simulink model "couplage_simulation"  (R2020a)
settings: Solver=VariableStepAuto  StartTime=0.0  StopTime=7  RelTol=1e-3
values from neighbouring files (symbols this model uses):
  cond_ini = [10; 10; 10; 0]    [bras.m]    (also in bras_espace.m = [10; 10; 10; 30]; bras_init.m = [10; 10; 10; 30]; init_simulation_couplage.m = [-pi/4; pi/4; -pi/4; 0])
  couples = [0; 0; 0; 0]    [init_simulation_couplage.m]
  inertie = [10; 10; 10]    [init_simulation_couplage.m]
  inertie_a = [0 0 0 0; 0 0 0 0; 0 0 0 0; 0 0 0 0]    [init_simulation_couplage.m]
  parametres = [m1; m2; m3; L1; L2; L3; l1; l2; l3; L0]    [init_simulation_couplage.m]
settings Model: Creator=loloche  LastModifiedBy=loloche

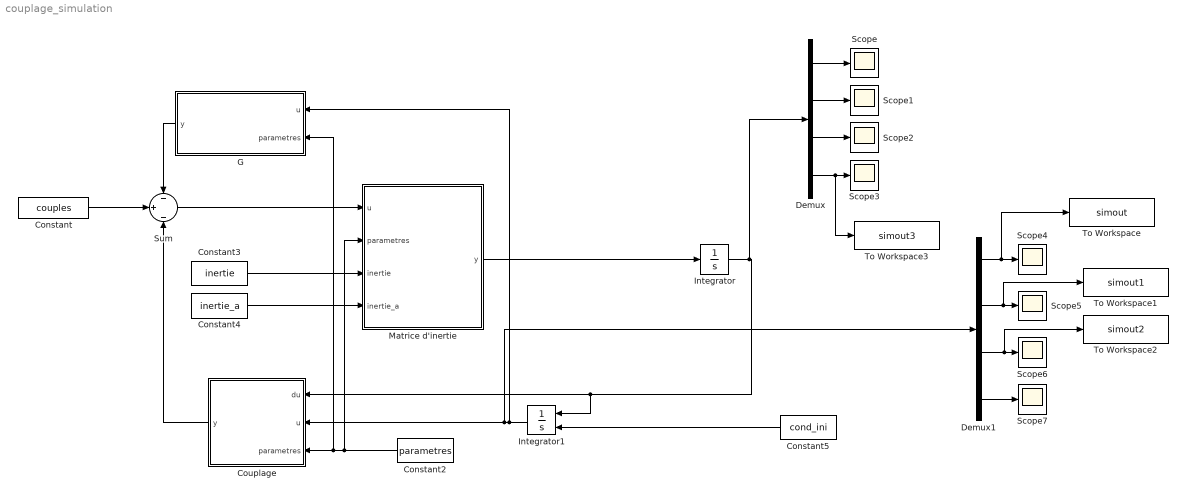
== system couplage_simulation ==
  Constant : Constant  Value=couples
  Constant2 : Constant  Value=parametres
  Constant3 : Constant  Value=inertie
  Constant4 : Constant  Value=inertie_a
  Constant5 : Constant  Value=cond_ini
  Couplage : MATLAB Function  TreatAsAtomicUnit=on
  Demux : Demux
  Demux1 : Demux
  G : MATLAB Function  TreatAsAtomicUnit=on
  Integrator : Integrator
  Integrator1 : Integrator  InitialConditionSource=external
  Matrice d'inertie : MATLAB Function  TreatAsAtomicUnit=on
  Scope{,1..7} (8 alike) : Scope
  Sum : Sum  Inputs=-|+|-
  To Workspace : ToWorkspace  VariableName=simout  SaveFormat=Structure With Time  SampleTime=-1
  To Workspace1 : ToWorkspace  VariableName=simout1  SaveFormat=Structure With Time  SampleTime=-1
  To Workspace2 : ToWorkspace  VariableName=simout2  SaveFormat=Structure With Time  SampleTime=-1
  To Workspace3 : ToWorkspace  VariableName=simout3  SaveFormat=Structure With Time  SampleTime=-1
  wires:
  Demux/1 -> Scope/1
  Demux/2 -> Scope1/1
  Demux/3 -> Scope2/1
  Constant/1 -> Sum/2
  G/1(y) -> Sum/1
  Couplage/1(y) -> Sum/3
  Matrice d'inertie/1(y) -> Integrator/1
  Integrator/1 -> Demux/1, Integrator1/1, Couplage/1(du)
  Constant5/1 -> Integrator1/2
  Integrator1/1 -> G/1(u), Couplage/2(u), Demux1/1
  Sum/1 -> Matrice d'inertie/1(u)
  Constant2/1 -> Matrice d'inertie/2(parametres), G/2(parametres), Couplage/3(parametres)
  Constant3/1 -> Matrice d'inertie/3(inertie)
  Constant4/1 -> Matrice d'inertie/4(inertie_a)
  Demux1/2 -> To Workspace1/1, Scope5/1
  Demux1/1 -> To Workspace/1, Scope4/1
  Demux/4 -> To Workspace3/1, Scope3/1
  Demux1/4 -> Scope7/1
  Demux1/3 -> To Workspace2/1, Scope6/1

== matlab function couplage_simulation/Matrice d'inertie ==
  data: u input; y output; parametres input; inertie input; inertie_a input
function y = fcn(u, parametres, inertie, inertie_a)
L1= parametres(4); %longueur bras
l1 = parametres(7); %distance centre inertie
L2 =parametres(5);
l2 = parametres(8);
m1 = parametres(1); %masse
m2 = parametres(2);
m3 = parametres(3);
L3 = parametres(6); %lamdba pour t=0
l3 = parametres(9);
ZZ1 = inertie(1);
ZZ2 = inertie(2);
ZZ3 = inertie(3);

theta1 = u(1);
theta2 = u(2);
theta3 = u(3);

A11 = ZZ1 + ZZ2 + m1*11*l1 + m2*(L1*L1 + l2*l2 + 2*L1*l2*cos(theta2));
A12 = ZZ2 + m2*(L1*l2*cos(theta2)+ l2*l2);
A21 = A12;
A22 = ZZ2 + m2*l2*l2;
A33 = ZZ3 + m3*l3*l2;
D = min([A11, A22, A33])*10^-4 


A = [A11 A12 0 0; A21 A22 0 0; 0 0 A33 0; 0 0 0 D];
M = A + inertie_a;

y = M\u;

== matlab function couplage_simulation/Couplage ==
  data: du input; u input; y output; parametres input
function y = fcn(du, u, parametres)

m1 = parametres(1);
m2 = parametres(2);
L1 = parametres(4);
L2 = parametres(5);
l1 = parametres(7);
l2= parametres(8);
L0 = parametres(10);

theta1 = u(1);
theta2 = u(2);
theta3 = u(3);

dtheta1 = du(1);
dtheta2 = du(2);

C11 = -m2*l2*L1*sin(theta2)*dtheta2;
C12 = -m2*l2*L1*sin(theta2 + theta1)*(dtheta2 + dtheta1);
C21= m2*l2*L1*sin(theta2)*dtheta1;
C22= 0;
C33= 0;

%Vecteurs directeurs
iz = [0 0 1];
r1 = [cos(theta1) sin(theta1) 0];
r2 = [cos(theta1 + theta2) sin(theta1 + theta2) 0];
r3 = [cos(theta3) sin(theta3) 0];

%Produits scalaires
r1r2 = dot(r1,r2);
r1r3 = dot(r1,r3);
r2r3 = dot(r2,r3);

%Produits vectoriels
iz_r1 = cross(iz,r1);
iz_r2 = cross(iz,r2);
iz_r3 = cross(iz,r3);

%Contrainte type pivot-glissière
A = dot(L1*iz_r1 + L2*iz_r2,iz_r3);
B = dot(L2*iz_r2,iz_r3);
C = -(L1*r1r3 + L2*r2r3 - cos(theta3));


%A = -L1*(sin(theta1)*sin(theta3) + cos(theta1)*cos(theta3))-L2*(sin(theta1+theta2)*sin(theta3)+cos(theta1+theta2)*cos(theta3));
%B = -L2*(sin(theta1+theta2)*sin(theta3)+cos(theta1+theta2)*cos(theta3));
%C = L1*cos(theta3-theta1) + L2*cos(theta3-theta2-theta1) - L0*cos(theta3);

mat = [C11 C12 0 -A; C21 C22 0 -B; 0 0 C33 -C; A B C 0];

mat_ex = mat(1:3,1:3);
y = mat*du;

== matlab function couplage_simulation/G ==
  data: u input; y output; parametres input
function y = fcn(u, parametres)

m1 = parametres(1);
m2 = parametres(2);
m3 = parametres(3);

L1 = parametres(4);
L2 = parametres(5);
l1 = parametres(7);
l2 = parametres(8);
l3 = parametres(9);

theta1 = u(1);
theta2 = u(2);
theta3 = u(3);

g=9.81;

G1 = cos(theta1)*(m1*l1*g + m2*L1*g)+m2*l2*g*cos(theta1 + theta2);
G2 = m2*l2*g*cos(theta1 +theta2);
G3 = m3*l3*g*cos(theta3);

y = [G1; G2; G3; 0];
